simulink model "FourRigidBarsAug"  (R2025b)
settings: Solver=VariableStepAuto  StartTime=0.0  StopTime=10.0  RelTol=1e-3
undefined symbols (not defined in the file): I1_G, I2_G, I3_G, Ignew, InvDynAug, Jr, l1, l2, l3, m1, m2, m3, ra_norm, sig4, Theta, uss
libraries: RCTblocks x99
(part 1 of 2)
settings Model: Creator=d.alazard  LastModifiedBy=andre
settings SolverCC: AlgebraicLoopSolver=TrustRegion
settings OptimizationCC: DefaultParameterBehavior=Inlined  BufferReuse=off
settings DebuggingCC: AlgebraicLoopMsg=none  UnconnectedInputMsg=warning  UnconnectedOutputMsg=warning  UnconnectedLineMsg=warning  InitInArrayFormatMsg=none
settings ModelReferenceCC: EnableRefExpFcnMdlSchedulingChecks=on
settings RTWCC: GPUComputeCapability=3.5  DLArmComputeVersion=19.05

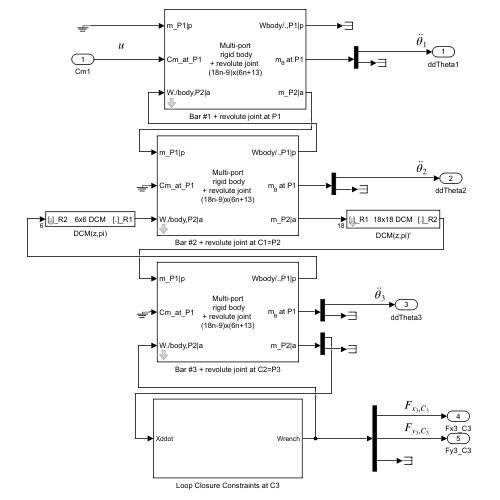
[thumbnail: Simulink's stored preview of the top-level diagram]
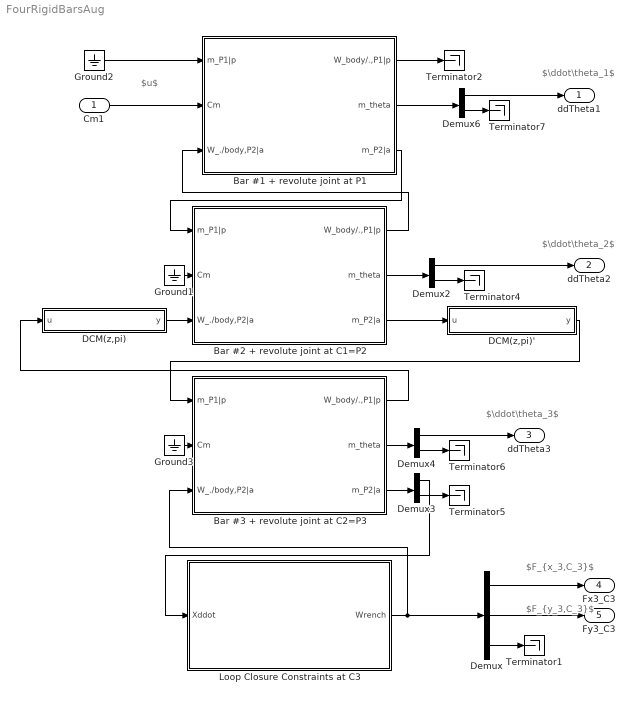
== system FourRigidBarsAug ==
  note: $F_{x_3,C_3}$
  note: $\ddot\theta_1$
  note: $u$
  note: $\ddot\theta_2$
  note: $\ddot\theta_3$
  note: $F_{y_3,C_3}$
  Cm1 : Inport
  Bar #1 + revolute joint at P1 : Subsystem  mask(Multi-port rigid body with revolute joint (18n-9)x(6n+15)){m=m1, Ig=I1_G, OG=[l1/2;0;0], n=2, OP1=[0;0;0], OP2=[l1;0;0], OP3=[0;0;0.25], OP4=[0;12;0], OP5=[0;0;0], ra=[0;0;1], theta=Theta}
      mask prompts: m "Mass (kg)"; Ig "Inertia at G in Ra (kg.m^2)"; OG "OG (3x1 vector in Ra)  (m)"; n "n (number of connection points)"; OP1 "OP1 (3x1 vector in Ra) (m)"; OP2 "OP2 (3x1 vector in Ra) (m)"; OP3 "OP3 (3x1 vector in Ra) (m)"; OP4 "OP4 (3x1 vector in Ra) (m)"; OP5 "OP5 (3x1 vector in Ra) (m)"; ra "ra (joint axis) (3x1 vector)"; theta "Angular configuration (rad)"
      mask help:
      | Computes the (18n-9)x(6n+13) model :
      | - 6x18 transfer from the motion vector to the wrench applied by this body to a parent body at port P1 through a revolute joint,
      | - the 3x1 channel :
      |               * from  the  joint torque applied by the input (parent) shaft to the output (body) shaft
      |               * to the relative motion vector of the output shaft w.r.t the input shaft ([thetaddot;thetadot;theta]),
      | - (n-1) 18x6 transfers from the wrenches applied to this body to the motion vectors at ports P2,P3,..,
      |
      | Input/Output of port P1 are expressed in the parent frame Rp
      | Input/Output of ports P2,P3,... are expressed in the body frame Ra.
      |
      | O: the body reference point
      | G: the center of mass
      | Pi (i=1:n): the n given connection points or ports (n<6).
      | ra: direction of the revolute joint in the Rp (or Ra)
      | theta: angular configuration of the joint (Ra is obtained from Rp by a rotation of theta around ra).
      |
      | All parameters must be expressed in the body frame Ra.
      | Each parameter can be an uncertain parameter declared with the function ureal (except ra)
      |
      | Rk: if "theta" field is: ureal('NAME',0,'Range',[-pi pi])
      | then, ULINEARIZE will provide a model involving the block named "tan_NAME_div4";
      mask init:
      | MultiPortRigidBodyRevAug
      mask Help: web('DocMultiportRigidBodyRevolute.html','-browser')
      mask TypeOptions n: 1 | 2 | 3 | 4 | 5
      mask DialogControl ParameterGroupVar Prompt: Rigid body parameter
      mask DialogControl port1 Prompt: #1
      mask DialogControl port2 Prompt: #2
      mask DialogControl port3 Prompt: #3
      mask DialogControl port4 Prompt: #4
      mask DialogControl port5 Prompt: #5
      mask DialogControl JointParameters Prompt: Revolute joint parameters
      mask Display:
      | disp('Multi-port\n rigid body\n+ revolute joint \n(18n-9)x(6n+13)')
      | 
      | port_label('input', 1,'m_P1|p')
      | port_label('output',1,'Wbody/.,P1|p')
      | port_label('input', 2,'Cm_at_P1')
      | port_label('output',2,'m_\theta at P1','interpreter','tex')
      | 
      | if n>1
      |     for i=2:n
      |         port_label('input', i+1,['W./body,P',num2str(i),'|a'])
      |         port_label('output',i+1,['m_P',num2str(i),'|a'])
      |     end
      | end
  Bar #2 + revolute joint at C1=P2 : Subsystem  mask(Multi-port rigid body with revolute joint (18n-9)x(6n+15)){m=m2, Ig=I2_G, OG=[l2/2;0;0], n=2, OP1=[0;0;0], OP2=[l2;0;0], OP3=[0;0;0.25], OP4=[0;12;0], OP5=[0;0;0], ra=[0;0;-1], theta=Theta}
      mask prompts: m "Mass (kg)"; Ig "Inertia at G in Ra (kg.m^2)"; OG "OG (3x1 vector in Ra)  (m)"; n "n (number of connection points)"; OP1 "OP1 (3x1 vector in Ra) (m)"; OP2 "OP2 (3x1 vector in Ra) (m)"; OP3 "OP3 (3x1 vector in Ra) (m)"; OP4 "OP4 (3x1 vector in Ra) (m)"; OP5 "OP5 (3x1 vector in Ra) (m)"; ra "ra (joint axis) (3x1 vector)"; theta "Angular configuration (rad)"
      mask help:
      | Computes the (18n-9)x(6n+13) model :
      | - 6x18 transfer from the motion vector to the wrench applied by this body to a parent body at port P1 through a revolute joint,
      | - the 3x1 channel :
      |               * from  the  joint torque applied by the input (parent) shaft to the output (body) shaft
      |               * to the relative motion vector of the output shaft w.r.t the input shaft ([thetaddot;thetadot;theta]),
      | - (n-1) 18x6 transfers from the wrenches applied to this body to the motion vectors at ports P2,P3,..,
      |
      | Input/Output of port P1 are expressed in the parent frame Rp
      | Input/Output of ports P2,P3,... are expressed in the body frame Ra.
      |
      | O: the body reference point
      | G: the center of mass
      | Pi (i=1:n): the n given connection points or ports (n<6).
      | ra: direction of the revolute joint in the Rp (or Ra)
      | theta: angular configuration of the joint (Ra is obtained from Rp by a rotation of theta around ra).
      |
      | All parameters must be expressed in the body frame Ra.
      | Each parameter can be an uncertain parameter declared with the function ureal (except ra)
      |
      | Rk: if "theta" field is: ureal('NAME',0,'Range',[-pi pi])
      | then, ULINEARIZE will provide a model involving the block named "tan_NAME_div4";
      mask init:
      | MultiPortRigidBodyRevAug
      mask Help: web('DocMultiportRigidBodyRevolute.html','-browser')
      mask TypeOptions n: 1 | 2 | 3 | 4 | 5
      mask DialogControl ParameterGroupVar Prompt: Rigid body parameter
      mask DialogControl port1 Prompt: #1
      mask DialogControl port2 Prompt: #2
      mask DialogControl port3 Prompt: #3
      mask DialogControl port4 Prompt: #4
      mask DialogControl port5 Prompt: #5
      mask DialogControl JointParameters Prompt: Revolute joint parameters
      mask Display:
      | disp('Multi-port\n rigid body\n+ revolute joint \n(18n-9)x(6n+13)')
      | 
      | port_label('input', 1,'m_P1|p')
      | port_label('output',1,'Wbody/.,P1|p')
      | port_label('input', 2,'Cm_at_P1')
      | port_label('output',2,'m_\theta at P1','interpreter','tex')
      | 
      | if n>1
      |     for i=2:n
      |         port_label('input', i+1,['W./body,P',num2str(i),'|a'])
      |         port_label('output',i+1,['m_P',num2str(i),'|a'])
      |     end
      | end
  Bar #3 + revolute joint at C2=P3 : Subsystem  mask(Multi-port rigid body with revolute joint (18n-9)x(6n+15)){m=m3, Ig=I3_G, OG=[l3/2;0;0], n=2, OP1=[0;0;0], OP2=[l3;0;0], OP3=[0;0;0.25], OP4=[0;12;0], OP5=[0;0;0], ra=[0;0;1], theta=Theta}
      mask prompts: m "Mass (kg)"; Ig "Inertia at G in Ra (kg.m^2)"; OG "OG (3x1 vector in Ra)  (m)"; n "n (number of connection points)"; OP1 "OP1 (3x1 vector in Ra) (m)"; OP2 "OP2 (3x1 vector in Ra) (m)"; OP3 "OP3 (3x1 vector in Ra) (m)"; OP4 "OP4 (3x1 vector in Ra) (m)"; OP5 "OP5 (3x1 vector in Ra) (m)"; ra "ra (joint axis) (3x1 vector)"; theta "Angular configuration (rad)"
      mask help:
      | Computes the (18n-9)x(6n+13) model :
      | - 6x18 transfer from the motion vector to the wrench applied by this body to a parent body at port P1 through a revolute joint,
      | - the 3x1 channel :
      |               * from  the  joint torque applied by the input (parent) shaft to the output (body) shaft
      |               * to the relative motion vector of the output shaft w.r.t the input shaft ([thetaddot;thetadot;theta]),
      | - (n-1) 18x6 transfers from the wrenches applied to this body to the motion vectors at ports P2,P3,..,
      |
      | Input/Output of port P1 are expressed in the parent frame Rp
      | Input/Output of ports P2,P3,... are expressed in the body frame Ra.
      |
      | O: the body reference point
      | G: the center of mass
      | Pi (i=1:n): the n given connection points or ports (n<6).
      | ra: direction of the revolute joint in the Rp (or Ra)
      | theta: angular configuration of the joint (Ra is obtained from Rp by a rotation of theta around ra).
      |
      | All parameters must be expressed in the body frame Ra.
      | Each parameter can be an uncertain parameter declared with the function ureal (except ra)
      |
      | Rk: if "theta" field is: ureal('NAME',0,'Range',[-pi pi])
      | then, ULINEARIZE will provide a model involving the block named "tan_NAME_div4";
      mask init:
      | MultiPortRigidBodyRevAug
      mask Help: web('DocMultiportRigidBodyRevolute.html','-browser')
      mask TypeOptions n: 1 | 2 | 3 | 4 | 5
      mask DialogControl ParameterGroupVar Prompt: Rigid body parameter
      mask DialogControl port1 Prompt: #1
      mask DialogControl port2 Prompt: #2
      mask DialogControl port3 Prompt: #3
      mask DialogControl port4 Prompt: #4
      mask DialogControl port5 Prompt: #5
      mask DialogControl JointParameters Prompt: Revolute joint parameters
      mask Display:
      | disp('Multi-port\n rigid body\n+ revolute joint \n(18n-9)x(6n+13)')
      | 
      | port_label('input', 1,'m_P1|p')
      | port_label('output',1,'Wbody/.,P1|p')
      | port_label('input', 2,'Cm_at_P1')
      | port_label('output',2,'m_\theta at P1','interpreter','tex')
      | 
      | if n>1
      |     for i=2:n
      |         port_label('input', i+1,['W./body,P',num2str(i),'|a'])
      |         port_label('output',i+1,['m_P',num2str(i),'|a'])
      |     end
      | end
  DCM(z,pi) : Subsystem  mask(6x6 Direction cosine matrix (DCM)){rot=[-1 0 0;0 -1 0;0 0 1], transp=off}
      mask prompts: rot "3x3 DCM"; transp "Matrix transposed"
      mask help:
      | For 6 d.o.f. body motion (3 translations and 3 rotations), this block Implement the 6x6 rotation matrix (or its transposed) for a given 3x3 DCM.
      |
      | Considering 2 frames R1 and  R2, the DCM between R1 and R2 is defined as the 3x3 matrix where each column is the component vector of each R2 orthogonal unit vector expressed in R1. Thus
      |
      |    [v]_R1 = DCM  * [v]_R2.
      mask init:
      | if transp,
      |     rot=rot';
      | end
      mask Help: web('Doc6dcm.html','-browser')
      mask Display:
      | disp('6x6 DCM')
      | if transp
      |     port_label('input', 1, '[.]_R1')
      |     port_label('output', 1, '[.]_R2')
      | else
      |     port_label('input', 1, '[.]_R2')
      |     port_label('output', 1, '[.]_R1')
      | end
  DCM(z,pi)' : Subsystem  mask(18x18 Direction cosine matrix (DCM)){rot=[-1 0 0;0 -1 0;0 0 1], transp=on}
      mask prompts: rot "3x3 DCM"; transp "Matrix transposed"
      mask help:
      | For 6 d.o.f. body motion vector (3 translations and 3 rotations, accelerations, velocities and positions), this block Implement the 18x18 rotation matrix (or its transposed) for a given 3x3 DCM.
      |
      | Considering 2 frames R1 and  R2, the DCM between R1 and R2 is defined as the 3x3 matrix where each column is the component vector of each R2 orthogonal unit vector expressed in R1. Thus
      |
      |    [v]_R1 = DCM  * [v]_R2.
      mask init:
      | if transp,
      |     rot=rot';
      | end
      mask Help: web('Doc18dcm.html','-browser')
      mask Display:
      | disp('18x18 DCM')
      | if transp
      |     port_label('input', 1, '[.]_R1')
      |     port_label('output', 1, '[.]_R2')
      | else
      |     port_label('input', 1, '[.]_R2')
      |     port_label('output', 1, '[.]_R1')
      | end
  Demux : Demux  Outputs=[1 1 4]
  Demux2 : Demux  Outputs=[1 2]
  Demux3 : Demux  Outputs=[6 12]
  Demux4 : Demux  Outputs=[1 2]
  Demux6 : Demux  Outputs=[1 2]
  Ground1 : Ground
  Ground2 : Ground
  Ground3 : Ground
  Loop Closure Constraints at C3 : Subsystem
  Terminator{1..2,4..7} (6 alike) : Terminator
  ddTheta1 : Outport
  ddTheta2 : Outport  Port=2
  ddTheta3 : Outport  Port=3
  Fx3_C3 : Outport  Port=4
  Fy3_C3 : Outport  Port=5
  wires:
  Bar #2 + revolute joint at C1=P2/1(W_body/.,P1|p) -> Bar #1 + revolute joint at P1/3(W_./body,P2|a)
  Cm1/1 -> Bar #1 + revolute joint at P1/2(Cm)
  Ground1/1 -> Bar #2 + revolute joint at C1=P2/2(Cm)
  Demux6/1 -> ddTheta1/1
  Demux2/1 -> ddTheta2/1
  DCM(z,pi)/1(y) -> Bar #2 + revolute joint at C1=P2/3(W_./body,P2|a)
  DCM(z,pi)'/1(y) -> Bar #3 + revolute joint at C2=P3/1(m_P1|p)
  Bar #3 + revolute joint at C2=P3/1(W_body/.,P1|p) -> DCM(z,pi)/1(u)
  Ground3/1 -> Bar #3 + revolute joint at C2=P3/2(Cm)
  Ground2/1 -> Bar #1 + revolute joint at P1/1(m_P1|p)
  Bar #1 + revolute joint at P1/1(W_body/.,P1|p) -> Terminator2/1
  Demux3/1 -> Loop Closure Constraints at C3/1(Xddot)
  Loop Closure Constraints at C3/1(Wrench) -> Demux/1, Bar #3 + revolute joint at C2=P3/3(W_./body,P2|a)
  Demux/3 -> Terminator1/1
  Demux/1 -> Fx3_C3/1
  Demux/2 -> Fy3_C3/1
  Bar #2 + revolute joint at C1=P2/2(m_theta) -> Demux2/1
  Demux2/2 -> Terminator4/1
  Demux4/2 -> Terminator6/1
  Bar #3 + revolute joint at C2=P3/2(m_theta) -> Demux4/1
  Demux3/2 -> Terminator5/1
  Bar #3 + revolute joint at C2=P3/3(m_P2|a) -> Demux3/1
  Demux4/1 -> ddTheta3/1
  Demux6/2 -> Terminator7/1
  Bar #1 + revolute joint at P1/2(m_theta) -> Demux6/1
  Bar #1 + revolute joint at P1/3(m_P2|a) -> Bar #2 + revolute joint at C1=P2/1(m_P1|p)
  Bar #2 + revolute joint at C1=P2/3(m_P2|a) -> DCM(z,pi)'/1(u)

== system FourRigidBarsAug/Bar #1 + revolute joint at P1 ==
  m_P1|p : Inport
  Cm : Inport  Port=2
  W_./body,P2|a : Inport  Port=3
  Multi port rigid body : Subsystem  mask(Multi-port rigid body (6nx6n)){m=m, Ig=Ignew, OG=OG, n=2, numinv=1, OP1=[0;0;0], OP2=[l1;0;0], OP3=[0;0;0.25], OP4=[0;12;0], OP5=[0;0;0]}
      mask prompts: m "Mass (Kg)"; Ig "Inertia (at G, Kg m^2)"; OG "OG (3x1 vector, m)"; n "Number of ports"; numinv "Port to be inverted"; OP1 "OP1 (3x1 vector, m)"; OP2 "OP2 (3x1 vector, m)"; OP3 "OP3 (3x1 vector, m)"; OP4 "OP4 (3x1 vector, m)"; OP5 "OP5 (3x1 vector,m)"
      mask help:
      | 6nx6n dynamic model of a rigid body at n given points (ports) between wrenches applied at the n points (input) and acceleration twists at these points (output).
      |
      | 0: the reference point
      | G: the center of mass
      | Pi (i=1:n): the n given connection points (n<6).
      |
      | All parameters are expressed in the body frame.
      | Each parameter can be an uncertain parameter declared with "ureal"
      |
      | The 6x6 channel associated to one port can be inverted: then the input of this channel is the acceleration twist imposed at this point and the output is the wrench applied by this body.
      mask init:
      | MultiPortRigidBodyAug
      mask Help: web('Docmultiportrigidbody.html','-browser')
      mask TypeOptions n: 1 | 2 | 3 | 4 | 5
      mask TypeOptions numinv: 1 | 2 | 3 | 4 | 5
      mask DialogControl ParameterGroupVar Prompt: Main parameters
      mask DialogControl port1 Prompt: Port #1
      mask DialogControl port2 Prompt: #2
      mask DialogControl port3 Prompt: #3
      mask DialogControl port4 Prompt: #4
      mask DialogControl port5 Prompt: #5
      mask Display:
      | disp('Multi-port\n rigid body\n [18(n-1)+6]x[6(n-1)+18])')
      | if n==1,
      |     if numinv==1,
      |         port_label('input', 1,'m_P')
      |         port_label('output',1,'W_body/.,P')
      |     else
      |         port_label('input', 1,'W_./body,P')
      |         port_label('output',1,'m_P')
      |     end
      | else
      |     for ii=1:n
      |         if numinv==ii,
      |             port_label('output',ii,['W_body/.,P',num2str(ii)])
      |             port_label('input', ii,['m_P',num2str(ii)])
      |         else
      |             port_label('input', ii,['W_./body,P',num2str(ii)])
      |             port_label('output',ii,['m_P',num2str(ii)])
      |         end
      |     end
      | end
  Revolute joint + configuration : Subsystem  mask(Revolute joint){ra=ra_norm, Jr=Jr, theta=theta}
      mask prompts: ra "Direction of the joint in the local frame (3x1 vector)"; Jr "Rotor inertia (kg.m^2)"; theta "Angular configuration (rad)"
      mask help:
      | This block implement the TITOP model of of a revolute joint.
      | The last channel is the transfer between the torque applied inside the joint by the input shaft to the output shaft and the relative angular acceleration of the output shaft w.r.t the input shaft.
      |
      | Angular configuration can be a vayring parameter: Ex:
      | ureal('NAME',0,'Range',[-pi pi])
      |
      | Then, ULINEARIZE will provide a model involving the block named "tan_NAME_div4";
      mask init:
      | pass=ra2DCMi(ra);
      | ran=[ra(1);ra(2);ra(3)]/norm(ra);
      mask Help: web('DocRevoluteJoint_configuration.html','-browser')
      mask Display:
      | disp('Revolute joint\nTITOP model\n+ angle configuration')
      | port_label('input', 1, 'W_./r_out|a')
      | port_label('output', 1, 'm_out|a')
      | port_label('input', 2, 'm_in|p')
      | port_label('output', 2, 'W_r_in/.|p')
      | port_label('input', 3, 'Cm')
      | port_label('output', 3, 'm_\theta','interpreter','tex')
  W_body/.,P1|p : Outport  VectorParamsAs1DForOutWhenUnconnected=off
  m_theta : Outport  Port=2  VectorParamsAs1DForOutWhenUnconnected=off
  m_P2|a : Outport  Port=3
  wires:
  Revolute joint + configuration/1(m_out|a) -> Multi port rigid body/1(in1)
  Multi port rigid body/1(out1) -> Revolute joint + configuration/1(W_./r_out|a)
  m_P1|p/1 -> Revolute joint + configuration/2(m_in|p)
  Cm/1 -> Revolute joint + configuration/3(Cm)
  Revolute joint + configuration/2(W_r_in/.|p) -> W_body/.,P1|p/1
  Revolute joint + configuration/3(m_theta) -> m_theta/1
  W_./body,P2|a/1 -> Multi port rigid body/2(in2)
  Multi port rigid body/2(out2) -> m_P2|a/1

== system FourRigidBarsAug/Bar #2 + revolute joint at C1=P2 ==
  m_P1|p : Inport
  Cm : Inport  Port=2
  W_./body,P2|a : Inport  Port=3
  Multi port rigid body : Subsystem  mask(Multi-port rigid body (6nx6n)){m=m, Ig=Ignew, OG=OG, n=2, numinv=1, OP1=[0;0;0], OP2=[l2;0;0], OP3=[0;0;0.25], OP4=[0;12;0], OP5=[0;0;0]}
      mask prompts: m "Mass (Kg)"; Ig "Inertia (at G, Kg m^2)"; OG "OG (3x1 vector, m)"; n "Number of ports"; numinv "Port to be inverted"; OP1 "OP1 (3x1 vector, m)"; OP2 "OP2 (3x1 vector, m)"; OP3 "OP3 (3x1 vector, m)"; OP4 "OP4 (3x1 vector, m)"; OP5 "OP5 (3x1 vector,m)"
      mask help:
      | 6nx6n dynamic model of a rigid body at n given points (ports) between wrenches applied at the n points (input) and acceleration twists at these points (output).
      |
      | 0: the reference point
      | G: the center of mass
      | Pi (i=1:n): the n given connection points (n<6).
      |
      | All parameters are expressed in the body frame.
      | Each parameter can be an uncertain parameter declared with "ureal"
      |
      | The 6x6 channel associated to one port can be inverted: then the input of this channel is the acceleration twist imposed at this point and the output is the wrench applied by this body.
      mask init:
      | MultiPortRigidBodyAug
      mask Help: web('Docmultiportrigidbody.html','-browser')
      mask TypeOptions n: 1 | 2 | 3 | 4 | 5
      mask TypeOptions numinv: 1 | 2 | 3 | 4 | 5
      mask DialogControl ParameterGroupVar Prompt: Main parameters
      mask DialogControl port1 Prompt: Port #1
      mask DialogControl port2 Prompt: #2
      mask DialogControl port3 Prompt: #3
      mask DialogControl port4 Prompt: #4
      mask DialogControl port5 Prompt: #5
      mask Display:
      | disp('Multi-port\n rigid body\n [18(n-1)+6]x[6(n-1)+18])')
      | if n==1,
      |     if numinv==1,
      |         port_label('input', 1,'m_P')
      |         port_label('output',1,'W_body/.,P')
      |     else
      |         port_label('input', 1,'W_./body,P')
      |         port_label('output',1,'m_P')
      |     end
      | else
      |     for ii=1:n
      |         if numinv==ii,
      |             port_label('output',ii,['W_body/.,P',num2str(ii)])
      |             port_label('input', ii,['m_P',num2str(ii)])
      |         else
      |             port_label('input', ii,['W_./body,P',num2str(ii)])
      |             port_label('output',ii,['m_P',num2str(ii)])
      |         end
      |     end
      | end
  Revolute joint + configuration : Subsystem  mask(Revolute joint){ra=ra_norm, Jr=Jr, theta=theta}
      mask prompts: ra "Direction of the joint in the local frame (3x1 vector)"; Jr "Rotor inertia (kg.m^2)"; theta "Angular configuration (rad)"
      mask help:
      | This block implement the TITOP model of of a revolute joint.
      | The last channel is the transfer between the torque applied inside the joint by the input shaft to the output shaft and the relative angular acceleration of the output shaft w.r.t the input shaft.
      |
      | Angular configuration can be a vayring parameter: Ex:
      | ureal('NAME',0,'Range',[-pi pi])
      |
      | Then, ULINEARIZE will provide a model involving the block named "tan_NAME_div4";
      mask init:
      | pass=ra2DCMi(ra);
      | ran=[ra(1);ra(2);ra(3)]/norm(ra);
      mask Help: web('DocRevoluteJoint_configuration.html','-browser')
      mask Display:
      | disp('Revolute joint\nTITOP model\n+ angle configuration')
      | port_label('input', 1, 'W_./r_out|a')
      | port_label('output', 1, 'm_out|a')
      | port_label('input', 2, 'm_in|p')
      | port_label('output', 2, 'W_r_in/.|p')
      | port_label('input', 3, 'Cm')
      | port_label('output', 3, 'm_\theta','interpreter','tex')
  W_body/.,P1|p : Outport  VectorParamsAs1DForOutWhenUnconnected=off
  m_theta : Outport  Port=2  VectorParamsAs1DForOutWhenUnconnected=off
  m_P2|a : Outport  Port=3
  wires:
  Revolute joint + configuration/1(m_out|a) -> Multi port rigid body/1(in1)
  Multi port rigid body/1(out1) -> Revolute joint + configuration/1(W_./r_out|a)
  m_P1|p/1 -> Revolute joint + configuration/2(m_in|p)
  Cm/1 -> Revolute joint + configuration/3(Cm)
  Revolute joint + configuration/2(W_r_in/.|p) -> W_body/.,P1|p/1
  Revolute joint + configuration/3(m_theta) -> m_theta/1
  W_./body,P2|a/1 -> Multi port rigid body/2(in2)
  Multi port rigid body/2(out2) -> m_P2|a/1

== system FourRigidBarsAug/Bar #3 + revolute joint at C2=P3 ==
  m_P1|p : Inport
  Cm : Inport  Port=2
  W_./body,P2|a : Inport  Port=3
  Multi port rigid body : Subsystem  mask(Multi-port rigid body (6nx6n)){m=m, Ig=Ignew, OG=OG, n=2, numinv=1, OP1=[0;0;0], OP2=[l3;0;0], OP3=[0;0;0.25], OP4=[0;12;0], OP5=[0;0;0]}
      mask prompts: m "Mass (Kg)"; Ig "Inertia (at G, Kg m^2)"; OG "OG (3x1 vector, m)"; n "Number of ports"; numinv "Port to be inverted"; OP1 "OP1 (3x1 vector, m)"; OP2 "OP2 (3x1 vector, m)"; OP3 "OP3 (3x1 vector, m)"; OP4 "OP4 (3x1 vector, m)"; OP5 "OP5 (3x1 vector,m)"
      mask help:
      | 6nx6n dynamic model of a rigid body at n given points (ports) between wrenches applied at the n points (input) and acceleration twists at these points (output).
      |
      | 0: the reference point
      | G: the center of mass
      | Pi (i=1:n): the n given connection points (n<6).
      |
      | All parameters are expressed in the body frame.
      | Each parameter can be an uncertain parameter declared with "ureal"
      |
      | The 6x6 channel associated to one port can be inverted: then the input of this channel is the acceleration twist imposed at this point and the output is the wrench applied by this body.
      mask init:
      | MultiPortRigidBodyAug
      mask Help: web('Docmultiportrigidbody.html','-browser')
      mask TypeOptions n: 1 | 2 | 3 | 4 | 5
      mask TypeOptions numinv: 1 | 2 | 3 | 4 | 5
      mask DialogControl ParameterGroupVar Prompt: Main parameters
      mask DialogControl port1 Prompt: Port #1
      mask DialogControl port2 Prompt: #2
      mask DialogControl port3 Prompt: #3
      mask DialogControl port4 Prompt: #4
      mask DialogControl port5 Prompt: #5
      mask Display:
      | disp('Multi-port\n rigid body\n [18(n-1)+6]x[6(n-1)+18])')
      | if n==1,
      |     if numinv==1,
      |         port_label('input', 1,'m_P')
      |         port_label('output',1,'W_body/.,P')
      |     else
      |         port_label('input', 1,'W_./body,P')
      |         port_label('output',1,'m_P')
      |     end
      | else
      |     for ii=1:n
      |         if numinv==ii,
      |             port_label('output',ii,['W_body/.,P',num2str(ii)])
      |             port_label('input', ii,['m_P',num2str(ii)])
      |         else
      |             port_label('input', ii,['W_./body,P',num2str(ii)])
      |             port_label('output',ii,['m_P',num2str(ii)])
      |         end
      |     end
      | end
  Revolute joint + configuration : Subsystem  mask(Revolute joint){ra=ra_norm, Jr=Jr, theta=theta}
      mask prompts: ra "Direction of the joint in the local frame (3x1 vector)"; Jr "Rotor inertia (kg.m^2)"; theta "Angular configuration (rad)"
      mask help:
      | This block implement the TITOP model of of a revolute joint.
      | The last channel is the transfer between the torque applied inside the joint by the input shaft to the output shaft and the relative angular acceleration of the output shaft w.r.t the input shaft.
      |
      | Angular configuration can be a vayring parameter: Ex:
      | ureal('NAME',0,'Range',[-pi pi])
      |
      | Then, ULINEARIZE will provide a model involving the block named "tan_NAME_div4";
      mask init:
      | pass=ra2DCMi(ra);
      | ran=[ra(1);ra(2);ra(3)]/norm(ra);
      mask Help: web('DocRevoluteJoint_configuration.html','-browser')
      mask Display:
      | disp('Revolute joint\nTITOP model\n+ angle configuration')
      | port_label('input', 1, 'W_./r_out|a')
      | port_label('output', 1, 'm_out|a')
      | port_label('input', 2, 'm_in|p')
      | port_label('output', 2, 'W_r_in/.|p')
      | port_label('input', 3, 'Cm')
      | port_label('output', 3, 'm_\theta','interpreter','tex')
  W_body/.,P1|p : Outport  VectorParamsAs1DForOutWhenUnconnected=off
  m_theta : Outport  Port=2  VectorParamsAs1DForOutWhenUnconnected=off
  m_P2|a : Outport  Port=3
  wires:
  Revolute joint + configuration/1(m_out|a) -> Multi port rigid body/1(in1)
  Multi port rigid body/1(out1) -> Revolute joint + configuration/1(W_./r_out|a)
  m_P1|p/1 -> Revolute joint + configuration/2(m_in|p)
  Cm/1 -> Revolute joint + configuration/3(Cm)
  Revolute joint + configuration/2(W_r_in/.|p) -> W_body/.,P1|p/1
  Revolute joint + configuration/3(m_theta) -> m_theta/1
  W_./body,P2|a/1 -> Multi port rigid body/2(in2)
  Multi port rigid body/2(out2) -> m_P2|a/1

== system FourRigidBarsAug/DCM(z,pi) ==
  u : Inport  PortDimensions=6
  Demux : Demux  Outputs=[3 3]
  Mux : Mux  Inputs=[3 3]
  rotation : Gain  Gain=rot  Multiplication=Matrix(K*u) (u vector)
  translation : Gain  Gain=rot  Multiplication=Matrix(K*u) (u vector)
  y : Outport  VectorParamsAs1DForOutWhenUnconnected=off
  wires:
  rotation/1 -> Mux/2
  translation/1 -> Mux/1
  Demux/1 -> translation/1
  u/1 -> Demux/1
  Mux/1 -> y/1
  Demux/2 -> rotation/1

== system FourRigidBarsAug/DCM(z,pi)' ==
  u : Inport  PortDimensions=18
  Demux : Demux  Outputs=[3 3 3 3 3 3]
  Mux : Mux  Inputs=[3 3 3 3 3 3]
  rotation : Gain  Gain=rot  Multiplication=Matrix(K*u) (u vector)
  rotation1 : Gain  Gain=rot  Multiplication=Matrix(K*u) (u vector)
  rotation2 : Gain  Gain=rot  Multiplication=Matrix(K*u) (u vector)
  translation : Gain  Gain=rot  Multiplication=Matrix(K*u) (u vector)
  translation1 : Gain  Gain=rot  Multiplication=Matrix(K*u) (u vector)
  translation2 : Gain  Gain=rot  Multiplication=Matrix(K*u) (u vector)
  y : Outport  VectorParamsAs1DForOutWhenUnconnected=off
  wires:
  Demux/6 -> rotation2/1
  rotation2/1 -> Mux/6
  translation2/1 -> Mux/5
  Demux/5 -> translation2/1
  rotation1/1 -> Mux/4
  translation1/1 -> Mux/3
  Demux/3 -> translation1/1
  Demux/4 -> rotation1/1
  Demux/2 -> rotation/1
  Mux/1 -> y/1
  u/1 -> Demux/1
  Demux/1 -> translation/1
  translation/1 -> Mux/1
  rotation/1 -> Mux/2

== system FourRigidBarsAug/Loop Closure Constraints at C3 ==
  Xddot : Inport
  Demux : Demux  Outputs=6
  Ground{5..8} (4 alike) : Ground
  Mux : Mux  Inputs=6
  Terminator{1,3..5} (4 alike) : Terminator
  mx : Gain  Gain=-1e6
  my : Gain  Gain=-1e6
  Wrench : Outport
  wires:
  Ground7/1 -> Mux/5
  Ground6/1 -> Mux/4
  Xddot/1 -> Demux/1
  Demux/4 -> Terminator3/1
  Ground8/1 -> Mux/6
  Demux/6 -> Terminator5/1
  Demux/5 -> Terminator4/1
  mx/1 -> Mux/1
  Demux/3 -> Terminator1/1
  my/1 -> Mux/2
  Mux/1 -> Wrench/1
  Ground5/1 -> Mux/3
  Demux/1 -> mx/1
  Demux/2 -> my/1

== system FourRigidBarsAug/Bar #1 + revolute joint at P1/Multi port rigid body ==
  in1 : Inport  PortDimensions=18
  in2 : Inport  Port=2  PortDimensions=6
  Demux : Demux  Outputs=[ 6 18]
  Gain : RCTblocks/Uncertain State Space  Tag=USS  USystem=uss(InvDynAug)  UValue=[]  X0=[]  uX0=[]
  Mux : Mux  Inputs=[ 18 6]
  out1 : Outport
  out2 : Outport  Port=2
  wires:
  Demux/2 -> out2/1
  in2/1 -> Mux/2
  Demux/1 -> out1/1
  in1/1 -> Mux/1
  Gain/1 -> Demux/1
  Mux/1 -> Gain/1

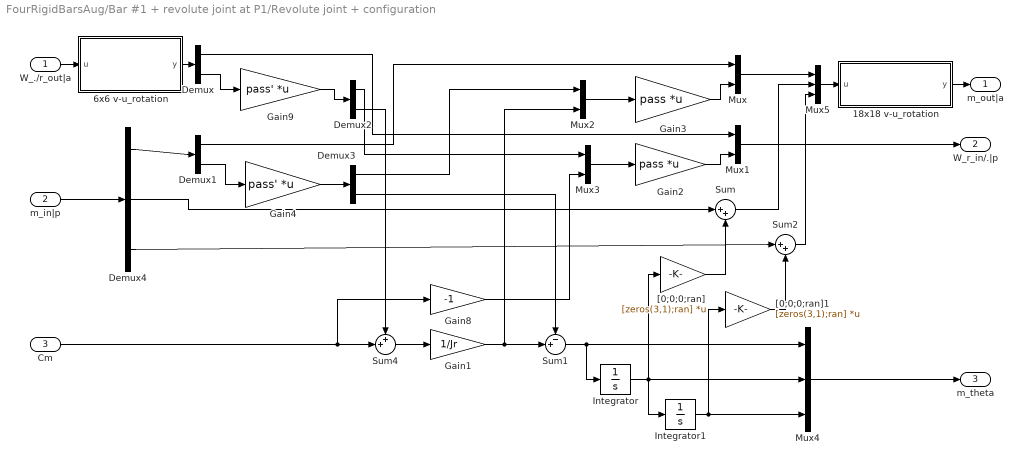
== system FourRigidBarsAug/Bar #1 + revolute joint at P1/Revolute joint + configuration ==
  W_./r_out|a : Inport  PortDimensions=6
  m_in|p : Inport  Port=2  PortDimensions=18
  Cm : Inport  Port=3  PortDimensions=1
  18x18 v-u_rotation : Subsystem  mask(18x18 rotation matrix (around a given axis)){ra=ra, theta=theta, transp=on}
      mask prompts: ra "Rotation axis (3x1 vector)"; theta "Angle (rad)"; transp "Matrix transposed"
      mask help:
      | For 6 d.o.f. body motion vector (3 translations and 3 rotations, acceleration velocities and positions), this block Implement the 18x18 rotation matrix (or its transposed)  for a given angle around a given axis.
      |
      | Angle  (rad) can be an uncertain parameter declared with "ureal" with mode 'Range'
      | Ex: ureal('NAME',0,'Range',[-pi pi])
      | Then, ULINEARIZE will provide a model involving the block named "tan_NAME_div4".
      mask init:
      | vUrotation3x3
      mask Help: web('Doc6vurotation.html','-browser')
      mask Display:
      | disp('v-rot\n18x18')
      | if transp
      |     port_label('input', 1, '[.]_R1')
      |     port_label('output', 1, '[.]_R2')
      | else
      |     port_label('input', 1, '[.]_R2')
      |     port_label('output', 1, '[.]_R1')
      | end
  6x6 v-u_rotation : Subsystem  mask(6x6 rotation matrix (around a given axis)){ra=ra, theta=theta, transp=off}
      mask prompts: ra "Rotation axis (3x1 vector)"; theta "Angle (rad)"; transp "Matrix transposed"
      mask help:
      | For 6 d.o.f. body motion (3 translations and 3 rotations), this block Implement the 6x6 rotation matrix (or its transposed) for a given angle around a given axis.
      |
      | Angle  (rad) can be an uncertain parameter declared with "ureal" with mode 'Range'
      | Ex: ureal('NAME',0,'Range',[-pi pi])
      | Then, ULINEARIZE will provide a model involving the block named "tan_NAME_div4".
      mask init:
      | vUrotation3x3
      mask Help: web('Doc6vurotation.html','-browser')
      mask Display:
      | disp('v-rot\n6x6')
      | if transp
      |     port_label('input', 1, '[.]_R1')
      |     port_label('output', 1, '[.]_R2')
      | else
      |     port_label('input', 1, '[.]_R2')
      |     port_label('output', 1, '[.]_R1')
      | end
  Demux : Demux  Outputs=[3 3]
  Demux1 : Demux  Outputs=[3 3]
  Demux2 : Demux  Outputs=[2 1]
  Demux3 : Demux  Outputs=[2 1]
  Demux4 : Demux  Outputs=[6 6 6]
  Gain1 : Gain  Gain=1/Jr
  Gain2 : Gain  Gain=pass  Multiplication=Matrix(K*u) (u vector)
  Gain3 : Gain  Gain=pass  Multiplication=Matrix(K*u) (u vector)
  Gain4 : Gain  Gain=pass'  Multiplication=Matrix(K*u) (u vector)
  Gain8 : Gain  Gain=-1
  Gain9 : Gain  Gain=pass'  Multiplication=Matrix(K*u) (u vector)
  Integrator : Integrator
  Integrator1 : Integrator
  Mux : Mux  Inputs=[3 3]
  Mux1 : Mux  Inputs=[3 3]
  Mux2 : Mux  Inputs=[2 1]
  Mux3 : Mux  Inputs=[2 1]
  Mux4 : Mux  Inputs=3
  Mux5 : Mux  Inputs=[6 6 6]
  Sum : Sum  Inputs=|++
  Sum1 : Sum  Inputs=-+|
  Sum2 : Sum  Inputs=|++
  Sum4 : Sum  Inputs=++|
  "[0;0;0;ran]" : Gain  Gain=[zeros(3,1);ran]  Multiplication=Matrix(K*u) (u vector)
  "[0;0;0;ran]1" : Gain  Gain=[zeros(3,1);ran]  Multiplication=Matrix(K*u) (u vector)
  m_out|a : Outport  VectorParamsAs1DForOutWhenUnconnected=off
  W_r_in/.|p : Outport  Port=2  VectorParamsAs1DForOutWhenUnconnected=off
  m_theta : Outport  Port=3  VectorParamsAs1DForOutWhenUnconnected=off
  wires:
  18x18 v-u_rotation/1(y) -> m_out|a/1
  6x6 v-u_rotation/1(y) -> Demux/1
  Demux3/1 -> Mux2/1
  Demux2/1 -> Mux3/1
  Gain8/1 -> Mux3/2
  Mux3/1 -> Gain2/1
  Gain4/1 -> Demux3/1
  Demux1/2 -> Gain4/1
  Mux2/1 -> Gain3/1
  Demux2/2 -> Sum4/1
  Gain9/1 -> Demux2/1
  Demux3/2 -> Sum1/1
  Gain3/1 -> Mux/2
  Sum4/1 -> Gain1/1
  Gain1/1 -> Sum1/2, Mux2/2
  Demux/2 -> Gain9/1
  Gain2/1 -> Mux1/2
  Demux/1 -> Mux1/1
  Cm/1 -> Sum4/2, Gain8/1
  Demux1/1 -> Mux/1
  Mux1/1 -> W_r_in/.|p/1
  W_./r_out|a/1 -> 6x6 v-u_rotation/1(u)
  Demux4/1 -> Demux1/1
  m_in|p/1 -> Demux4/1
  Integrator/1 -> "[0;0;0;ran]"/1, Mux4/2, Integrator1/1
  Mux4/1 -> m_theta/1
  Sum1/1 -> Integrator/1, Mux4/1
  Integrator1/1 -> "[0;0;0;ran]1"/1, Mux4/3
  "[0;0;0;ran]"/1 -> Sum/2
  "[0;0;0;ran]1"/1 -> Sum2/2
  Demux4/2 -> Sum/1
  Demux4/3 -> Sum2/1
  Mux/1 -> Mux5/1
  Mux5/1 -> 18x18 v-u_rotation/1(u)
  Sum/1 -> Mux5/2
  Sum2/1 -> Mux5/3

== system FourRigidBarsAug/Bar #2 + revolute joint at C1=P2/Multi port rigid body ==
  in1 : Inport  PortDimensions=18
  in2 : Inport  Port=2  PortDimensions=6
  Demux : Demux  Outputs=[ 6 18]
  Gain : RCTblocks/Uncertain State Space  Tag=USS  USystem=uss(InvDynAug)  UValue=[]  X0=[]  uX0=[]
  Mux : Mux  Inputs=[ 18 6]
  out1 : Outport
  out2 : Outport  Port=2
  wires:
  Mux/1 -> Gain/1
  Gain/1 -> Demux/1
  in1/1 -> Mux/1
  Demux/1 -> out1/1
  in2/1 -> Mux/2
  Demux/2 -> out2/1

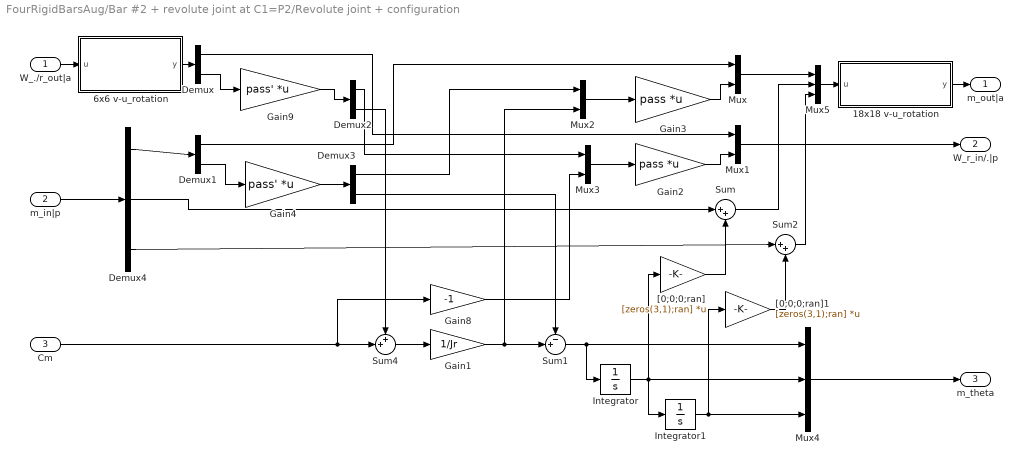
== system FourRigidBarsAug/Bar #2 + revolute joint at C1=P2/Revolute joint + configuration ==
  W_./r_out|a : Inport  PortDimensions=6
  m_in|p : Inport  Port=2  PortDimensions=18
  Cm : Inport  Port=3  PortDimensions=1
  18x18 v-u_rotation : Subsystem  mask(18x18 rotation matrix (around a given axis)){ra=ra, theta=theta, transp=on}
      mask prompts: ra "Rotation axis (3x1 vector)"; theta "Angle (rad)"; transp "Matrix transposed"
      mask help:
      | For 6 d.o.f. body motion vector (3 translations and 3 rotations, acceleration velocities and positions), this block Implement the 18x18 rotation matrix (or its transposed)  for a given angle around a given axis.
      |
      | Angle  (rad) can be an uncertain parameter declared with "ureal" with mode 'Range'
      | Ex: ureal('NAME',0,'Range',[-pi pi])
      | Then, ULINEARIZE will provide a model involving the block named "tan_NAME_div4".
      mask init:
      | vUrotation3x3
      mask Help: web('Doc6vurotation.html','-browser')
      mask Display:
      | disp('v-rot\n18x18')
      | if transp
      |     port_label('input', 1, '[.]_R1')
      |     port_label('output', 1, '[.]_R2')
      | else
      |     port_label('input', 1, '[.]_R2')
      |     port_label('output', 1, '[.]_R1')
      | end
  6x6 v-u_rotation : Subsystem  mask(6x6 rotation matrix (around a given axis)){ra=ra, theta=theta, transp=off}
      mask prompts: ra "Rotation axis (3x1 vector)"; theta "Angle (rad)"; transp "Matrix transposed"
      mask help:
      | For 6 d.o.f. body motion (3 translations and 3 rotations), this block Implement the 6x6 rotation matrix (or its transposed) for a given angle around a given axis.
      |
      | Angle  (rad) can be an uncertain parameter declared with "ureal" with mode 'Range'
      | Ex: ureal('NAME',0,'Range',[-pi pi])
      | Then, ULINEARIZE will provide a model involving the block named "tan_NAME_div4".
      mask init:
      | vUrotation3x3
      mask Help: web('Doc6vurotation.html','-browser')
      mask Display:
      | disp('v-rot\n6x6')
      | if transp
      |     port_label('input', 1, '[.]_R1')
      |     port_label('output', 1, '[.]_R2')
      | else
      |     port_label('input', 1, '[.]_R2')
      |     port_label('output', 1, '[.]_R1')
      | end
  Demux : Demux  Outputs=[3 3]
  Demux1 : Demux  Outputs=[3 3]
  Demux2 : Demux  Outputs=[2 1]
  Demux3 : Demux  Outputs=[2 1]
  Demux4 : Demux  Outputs=[6 6 6]
  Gain1 : Gain  Gain=1/Jr
  Gain2 : Gain  Gain=pass  Multiplication=Matrix(K*u) (u vector)
  Gain3 : Gain  Gain=pass  Multiplication=Matrix(K*u) (u vector)
  Gain4 : Gain  Gain=pass'  Multiplication=Matrix(K*u) (u vector)
  Gain8 : Gain  Gain=-1
  Gain9 : Gain  Gain=pass'  Multiplication=Matrix(K*u) (u vector)
  Integrator : Integrator
  Integrator1 : Integrator
  Mux : Mux  Inputs=[3 3]
  Mux1 : Mux  Inputs=[3 3]
  Mux2 : Mux  Inputs=[2 1]
  Mux3 : Mux  Inputs=[2 1]
  Mux4 : Mux  Inputs=3
  Mux5 : Mux  Inputs=[6 6 6]
  Sum : Sum  Inputs=|++
  Sum1 : Sum  Inputs=-+|
  Sum2 : Sum  Inputs=|++
  Sum4 : Sum  Inputs=++|
  "[0;0;0;ran]" : Gain  Gain=[zeros(3,1);ran]  Multiplication=Matrix(K*u) (u vector)
  "[0;0;0;ran]1" : Gain  Gain=[zeros(3,1);ran]  Multiplication=Matrix(K*u) (u vector)
  m_out|a : Outport  VectorParamsAs1DForOutWhenUnconnected=off
  W_r_in/.|p : Outport  Port=2  VectorParamsAs1DForOutWhenUnconnected=off
  m_theta : Outport  Port=3  VectorParamsAs1DForOutWhenUnconnected=off
  wires:
  Sum2/1 -> Mux5/3
  Sum/1 -> Mux5/2
  Mux5/1 -> 18x18 v-u_rotation/1(u)
  Mux/1 -> Mux5/1
  Demux4/3 -> Sum2/1
  Demux4/2 -> Sum/1
  "[0;0;0;ran]1"/1 -> Sum2/2
  "[0;0;0;ran]"/1 -> Sum/2
  Integrator1/1 -> Mux4/3, "[0;0;0;ran]1"/1
  Sum1/1 -> Mux4/1, Integrator/1
  Mux4/1 -> m_theta/1
  Integrator/1 -> Integrator1/1, Mux4/2, "[0;0;0;ran]"/1
  m_in|p/1 -> Demux4/1
  Demux4/1 -> Demux1/1
  W_./r_out|a/1 -> 6x6 v-u_rotation/1(u)
  Mux1/1 -> W_r_in/.|p/1
  Demux1/1 -> Mux/1
  Cm/1 -> Gain8/1, Sum4/2
  Demux/1 -> Mux1/1
  Gain2/1 -> Mux1/2
  Demux/2 -> Gain9/1
  Gain1/1 -> Mux2/2, Sum1/2
  Sum4/1 -> Gain1/1
  Gain3/1 -> Mux/2
  Demux3/2 -> Sum1/1
  Gain9/1 -> Demux2/1
  Demux2/2 -> Sum4/1
  Mux2/1 -> Gain3/1
  Demux1/2 -> Gain4/1
  Gain4/1 -> Demux3/1
  Mux3/1 -> Gain2/1
  Gain8/1 -> Mux3/2
  Demux2/1 -> Mux3/1
  Demux3/1 -> Mux2/1
  6x6 v-u_rotation/1(y) -> Demux/1
  18x18 v-u_rotation/1(y) -> m_out|a/1

== system FourRigidBarsAug/Bar #3 + revolute joint at C2=P3/Multi port rigid body ==
  in1 : Inport  PortDimensions=18
  in2 : Inport  Port=2  PortDimensions=6
  Demux : Demux  Outputs=[ 6 18]
  Gain : RCTblocks/Uncertain State Space  Tag=USS  USystem=uss(InvDynAug)  UValue=[]  X0=[]  uX0=[]
  Mux : Mux  Inputs=[ 18 6]
  out1 : Outport
  out2 : Outport  Port=2
  wires:
  Demux/2 -> out2/1
  in2/1 -> Mux/2
  Demux/1 -> out1/1
  in1/1 -> Mux/1
  Gain/1 -> Demux/1
  Mux/1 -> Gain/1

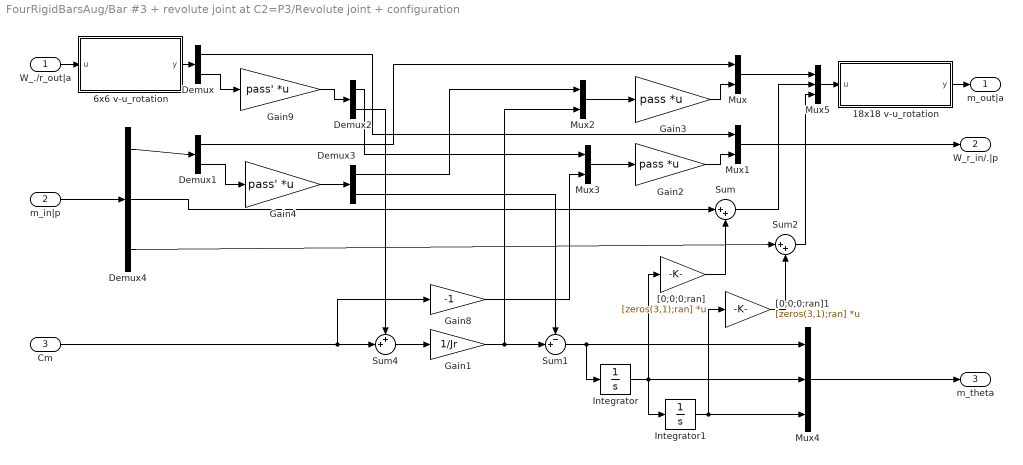
== system FourRigidBarsAug/Bar #3 + revolute joint at C2=P3/Revolute joint + configuration ==
  W_./r_out|a : Inport  PortDimensions=6
  m_in|p : Inport  Port=2  PortDimensions=18
  Cm : Inport  Port=3  PortDimensions=1
  18x18 v-u_rotation : Subsystem  mask(18x18 rotation matrix (around a given axis)){ra=ra, theta=theta, transp=on}
      mask prompts: ra "Rotation axis (3x1 vector)"; theta "Angle (rad)"; transp "Matrix transposed"
      mask help:
      | For 6 d.o.f. body motion vector (3 translations and 3 rotations, acceleration velocities and positions), this block Implement the 18x18 rotation matrix (or its transposed)  for a given angle around a given axis.
      |
      | Angle  (rad) can be an uncertain parameter declared with "ureal" with mode 'Range'
      | Ex: ureal('NAME',0,'Range',[-pi pi])
      | Then, ULINEARIZE will provide a model involving the block named "tan_NAME_div4".
      mask init:
      | vUrotation3x3
      mask Help: web('Doc6vurotation.html','-browser')
      mask Display:
      | disp('v-rot\n18x18')
      | if transp
      |     port_label('input', 1, '[.]_R1')
      |     port_label('output', 1, '[.]_R2')
      | else
      |     port_label('input', 1, '[.]_R2')
      |     port_label('output', 1, '[.]_R1')
      | end
  6x6 v-u_rotation : Subsystem  mask(6x6 rotation matrix (around a given axis)){ra=ra, theta=theta, transp=off}
      mask prompts: ra "Rotation axis (3x1 vector)"; theta "Angle (rad)"; transp "Matrix transposed"
      mask help:
      | For 6 d.o.f. body motion (3 translations and 3 rotations), this block Implement the 6x6 rotation matrix (or its transposed) for a given angle around a given axis.
      |
      | Angle  (rad) can be an uncertain parameter declared with "ureal" with mode 'Range'
      | Ex: ureal('NAME',0,'Range',[-pi pi])
      | Then, ULINEARIZE will provide a model involving the block named "tan_NAME_div4".
      mask init:
      | vUrotation3x3
      mask Help: web('Doc6vurotation.html','-browser')
      mask Display:
      | disp('v-rot\n6x6')
      | if transp
      |     port_label('input', 1, '[.]_R1')
      |     port_label('output', 1, '[.]_R2')
      | else
      |     port_label('input', 1, '[.]_R2')
      |     port_label('output', 1, '[.]_R1')
      | end
  Demux : Demux  Outputs=[3 3]
  Demux1 : Demux  Outputs=[3 3]
  Demux2 : Demux  Outputs=[2 1]
  Demux3 : Demux  Outputs=[2 1]
  Demux4 : Demux  Outputs=[6 6 6]
  Gain1 : Gain  Gain=1/Jr
  Gain2 : Gain  Gain=pass  Multiplication=Matrix(K*u) (u vector)
  Gain3 : Gain  Gain=pass  Multiplication=Matrix(K*u) (u vector)
  Gain4 : Gain  Gain=pass'  Multiplication=Matrix(K*u) (u vector)
  Gain8 : Gain  Gain=-1
  Gain9 : Gain  Gain=pass'  Multiplication=Matrix(K*u) (u vector)
  Integrator : Integrator
  Integrator1 : Integrator
  Mux : Mux  Inputs=[3 3]
  Mux1 : Mux  Inputs=[3 3]
  Mux2 : Mux  Inputs=[2 1]
  Mux3 : Mux  Inputs=[2 1]
  Mux4 : Mux  Inputs=3
  Mux5 : Mux  Inputs=[6 6 6]
  Sum : Sum  Inputs=|++
  Sum1 : Sum  Inputs=-+|
  Sum2 : Sum  Inputs=|++
  Sum4 : Sum  Inputs=++|
  "[0;0;0;ran]" : Gain  Gain=[zeros(3,1);ran]  Multiplication=Matrix(K*u) (u vector)
  "[0;0;0;ran]1" : Gain  Gain=[zeros(3,1);ran]  Multiplication=Matrix(K*u) (u vector)
  m_out|a : Outport  VectorParamsAs1DForOutWhenUnconnected=off
  W_r_in/.|p : Outport  Port=2  VectorParamsAs1DForOutWhenUnconnected=off
  m_theta : Outport  Port=3  VectorParamsAs1DForOutWhenUnconnected=off
  wires:
  18x18 v-u_rotation/1(y) -> m_out|a/1
  6x6 v-u_rotation/1(y) -> Demux/1
  Demux3/1 -> Mux2/1
  Demux2/1 -> Mux3/1
  Gain8/1 -> Mux3/2
  Mux3/1 -> Gain2/1
  Gain4/1 -> Demux3/1
  Demux1/2 -> Gain4/1
  Mux2/1 -> Gain3/1
  Demux2/2 -> Sum4/1
  Gain9/1 -> Demux2/1
  Demux3/2 -> Sum1/1
  Gain3/1 -> Mux/2
  Sum4/1 -> Gain1/1
  Gain1/1 -> Sum1/2, Mux2/2
  Demux/2 -> Gain9/1
  Gain2/1 -> Mux1/2
  Demux/1 -> Mux1/1
  Cm/1 -> Sum4/2, Gain8/1
  Demux1/1 -> Mux/1
  Mux1/1 -> W_r_in/.|p/1
  W_./r_out|a/1 -> 6x6 v-u_rotation/1(u)
  Demux4/1 -> Demux1/1
  m_in|p/1 -> Demux4/1
  Integrator/1 -> "[0;0;0;ran]"/1, Mux4/2, Integrator1/1
  Mux4/1 -> m_theta/1
  Sum1/1 -> Integrator/1, Mux4/1
  Integrator1/1 -> "[0;0;0;ran]1"/1, Mux4/3
  "[0;0;0;ran]"/1 -> Sum/2
  "[0;0;0;ran]1"/1 -> Sum2/2
  Demux4/2 -> Sum/1
  Demux4/3 -> Sum2/1
  Mux/1 -> Mux5/1
  Mux5/1 -> 18x18 v-u_rotation/1(u)
  Sum/1 -> Mux5/2
  Sum2/1 -> Mux5/3

== system FourRigidBarsAug/Bar #1 + revolute joint at P1/Revolute joint + configuration/18x18 v-u_rotation ==
  u : Inport  PortDimensions=18
  Demux : Demux  Outputs=[3 3 3 3 3 3]
  Mux : Mux  Inputs=[3 3 3 3 3 3]
  Subsystem : Subsystem
  Subsystem1 : Subsystem
  Subsystem2 : Subsystem
  Subsystem3 : Subsystem
  Subsystem4 : Subsystem
  Subsystem5 : Subsystem
  y : Outport  VectorParamsAs1DForOutWhenUnconnected=off
  wires:
  Subsystem1/1(Out1) -> Mux/2
  Subsystem/1(Out1) -> Mux/1
  Demux/2 -> Subsystem1/1(In1)
  Demux/1 -> Subsystem/1(In1)
  u/1 -> Demux/1
  Mux/1 -> y/1
  Demux/3 -> Subsystem2/1(In1)
  Subsystem2/1(Out1) -> Mux/3
  Demux/4 -> Subsystem3/1(In1)
  Subsystem3/1(Out1) -> Mux/4
  Demux/5 -> Subsystem4/1(In1)
  Subsystem4/1(Out1) -> Mux/5
  Demux/6 -> Subsystem5/1(In1)
  Subsystem5/1(Out1) -> Mux/6

== system FourRigidBarsAug/Bar #1 + revolute joint at P1/Revolute joint + configuration/6x6 v-u_rotation ==
  u : Inport  PortDimensions=6
  Demux : Demux  Outputs=[3 3]
  Mux : Mux  Inputs=[3 3]
  Subsystem : Subsystem
  Subsystem1 : Subsystem
  y : Outport  VectorParamsAs1DForOutWhenUnconnected=off
  wires:
  Mux/1 -> y/1
  u/1 -> Demux/1
  Demux/1 -> Subsystem/1(In1)
  Demux/2 -> Subsystem1/1(In1)
  Subsystem/1(Out1) -> Mux/1
  Subsystem1/1(Out1) -> Mux/2

== system FourRigidBarsAug/Bar #2 + revolute joint at C1=P2/Revolute joint + configuration/18x18 v-u_rotation ==
  u : Inport  PortDimensions=18
  Demux : Demux  Outputs=[3 3 3 3 3 3]
  Mux : Mux  Inputs=[3 3 3 3 3 3]
  Subsystem : Subsystem
  Subsystem1 : Subsystem
  Subsystem2 : Subsystem
  Subsystem3 : Subsystem
  Subsystem4 : Subsystem
  Subsystem5 : Subsystem
  y : Outport  VectorParamsAs1DForOutWhenUnconnected=off
  wires:
  Subsystem5/1(Out1) -> Mux/6
  Demux/6 -> Subsystem5/1(In1)
  Subsystem4/1(Out1) -> Mux/5
  Demux/5 -> Subsystem4/1(In1)
  Subsystem3/1(Out1) -> Mux/4
  Demux/4 -> Subsystem3/1(In1)
  Subsystem2/1(Out1) -> Mux/3
  Demux/3 -> Subsystem2/1(In1)
  Mux/1 -> y/1
  u/1 -> Demux/1
  Demux/1 -> Subsystem/1(In1)
  Demux/2 -> Subsystem1/1(In1)
  Subsystem/1(Out1) -> Mux/1
  Subsystem1/1(Out1) -> Mux/2

== system FourRigidBarsAug/Bar #2 + revolute joint at C1=P2/Revolute joint + configuration/6x6 v-u_rotation ==
  u : Inport  PortDimensions=6
  Demux : Demux  Outputs=[3 3]
  Mux : Mux  Inputs=[3 3]
  Subsystem : Subsystem
  Subsystem1 : Subsystem
  y : Outport  VectorParamsAs1DForOutWhenUnconnected=off
  wires:
  Subsystem1/1(Out1) -> Mux/2
  Subsystem/1(Out1) -> Mux/1
  Demux/2 -> Subsystem1/1(In1)
  Demux/1 -> Subsystem/1(In1)
  u/1 -> Demux/1
  Mux/1 -> y/1

== system FourRigidBarsAug/Bar #3 + revolute joint at C2=P3/Revolute joint + configuration/18x18 v-u_rotation ==
  u : Inport  PortDimensions=18
  Demux : Demux  Outputs=[3 3 3 3 3 3]
  Mux : Mux  Inputs=[3 3 3 3 3 3]
  Subsystem : Subsystem
  Subsystem1 : Subsystem
  Subsystem2 : Subsystem
  Subsystem3 : Subsystem
  Subsystem4 : Subsystem
  Subsystem5 : Subsystem
  y : Outport  VectorParamsAs1DForOutWhenUnconnected=off
  wires:
  Subsystem1/1(Out1) -> Mux/2
  Subsystem/1(Out1) -> Mux/1
  Demux/2 -> Subsystem1/1(In1)
  Demux/1 -> Subsystem/1(In1)
  u/1 -> Demux/1
  Mux/1 -> y/1
  Demux/3 -> Subsystem2/1(In1)
  Subsystem2/1(Out1) -> Mux/3
  Demux/4 -> Subsystem3/1(In1)
  Subsystem3/1(Out1) -> Mux/4
  Demux/5 -> Subsystem4/1(In1)
  Subsystem4/1(Out1) -> Mux/5
  Demux/6 -> Subsystem5/1(In1)
  Subsystem5/1(Out1) -> Mux/6

== system FourRigidBarsAug/Bar #3 + revolute joint at C2=P3/Revolute joint + configuration/6x6 v-u_rotation ==
  u : Inport  PortDimensions=6
  Demux : Demux  Outputs=[3 3]
  Mux : Mux  Inputs=[3 3]
  Subsystem : Subsystem
  Subsystem1 : Subsystem
  y : Outport  VectorParamsAs1DForOutWhenUnconnected=off
  wires:
  Mux/1 -> y/1
  u/1 -> Demux/1
  Demux/1 -> Subsystem/1(In1)
  Demux/2 -> Subsystem1/1(In1)
  Subsystem/1(Out1) -> Mux/1
  Subsystem1/1(Out1) -> Mux/2

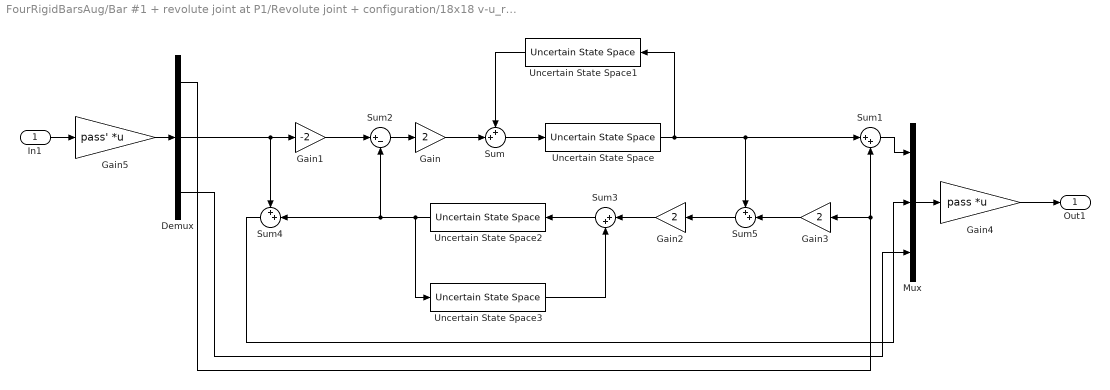
== system FourRigidBarsAug/Bar #1 + revolute joint at P1/Revolute joint + configuration/18x18 v-u_rotation/Subsystem ==
  In1 : Inport
  Demux : Demux  Outputs=3
  Gain : Gain  Gain=2
  Gain1 : Gain  Gain=-2
  Gain2 : Gain  Gain=2
  Gain3 : Gain  Gain=2
  Gain4 : Gain  Gain=pass  Multiplication=Matrix(K*u) (u vector)
  Gain5 : Gain  Gain=pass'  Multiplication=Matrix(K*u) (u vector)
  Mux : Mux  Inputs=3
  Sum : Sum  Inputs=++|
  Sum1 : Sum  Inputs=|++
  Sum2 : Sum  Inputs=|+-
  Sum3 : Sum  Inputs=|++
  Sum4 : Sum  Inputs=++|
  Sum5 : Sum  Inputs=++|
  Uncertain State Space{,1..3} (4 alike) : RCTblocks/Uncertain State Space  Tag=USS  USystem=uss(sig4)  UValue=[]  X0=[]  uX0=[]
  Out1 : Outport  VectorParamsAs1DForOutWhenUnconnected=off
  wires:
  Gain5/1 -> Demux/1
  Gain4/1 -> Out1/1
  Uncertain State Space3/1 -> Sum3/2
  Gain2/1 -> Sum3/1
  In1/1 -> Gain5/1
  Gain/1 -> Sum/2
  Uncertain State Space2/1 -> Uncertain State Space3/1, Sum4/2, Sum2/2
  Demux/1 -> Gain3/1, Sum1/2
  Demux/3 -> Mux/3
  Mux/1 -> Gain4/1
  Sum4/1 -> Mux/2
  Sum3/1 -> Uncertain State Space2/1
  Gain1/1 -> Sum2/1
  Uncertain State Space/1 -> Uncertain State Space1/1, Sum5/1, Sum1/1
  Gain3/1 -> Sum5/2
  Sum/1 -> Uncertain State Space/1
  Demux/2 -> Sum4/1, Gain1/1
  Uncertain State Space1/1 -> Sum/1
  Sum2/1 -> Gain/1
  Sum1/1 -> Mux/1
  Sum5/1 -> Gain2/1

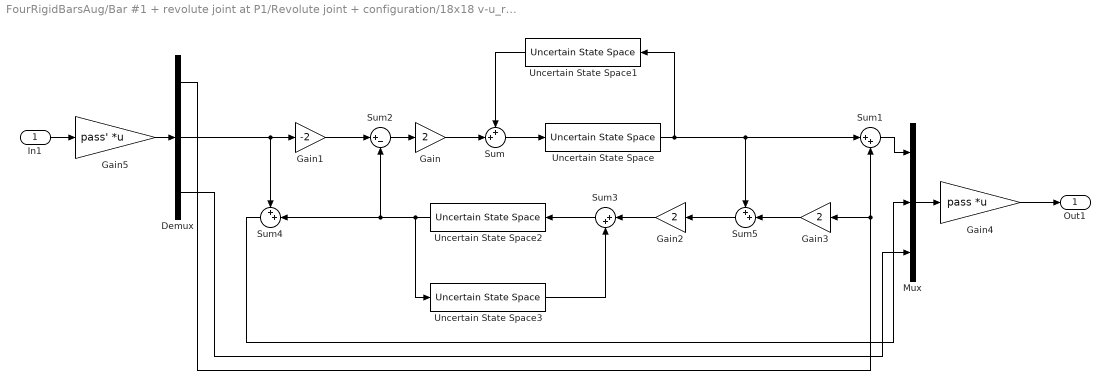
== system FourRigidBarsAug/Bar #1 + revolute joint at P1/Revolute joint + configuration/18x18 v-u_rotation/Subsystem1 ==
  In1 : Inport
  Demux : Demux  Outputs=3
  Gain : Gain  Gain=2
  Gain1 : Gain  Gain=-2
  Gain2 : Gain  Gain=2
  Gain3 : Gain  Gain=2
  Gain4 : Gain  Gain=pass  Multiplication=Matrix(K*u) (u vector)
  Gain5 : Gain  Gain=pass'  Multiplication=Matrix(K*u) (u vector)
  Mux : Mux  Inputs=3
  Sum : Sum  Inputs=++|
  Sum1 : Sum  Inputs=|++
  Sum2 : Sum  Inputs=|+-
  Sum3 : Sum  Inputs=|++
  Sum4 : Sum  Inputs=++|
  Sum5 : Sum  Inputs=++|
  Uncertain State Space{,1..3} (4 alike) : RCTblocks/Uncertain State Space  Tag=USS  USystem=uss(sig4)  UValue=[]  X0=[]  uX0=[]
  Out1 : Outport  VectorParamsAs1DForOutWhenUnconnected=off
  wires:
  Gain5/1 -> Demux/1
  Sum5/1 -> Gain2/1
  Sum1/1 -> Mux/1
  Sum2/1 -> Gain/1
  Uncertain State Space1/1 -> Sum/1
  Demux/2 -> Gain1/1, Sum4/1
  Sum/1 -> Uncertain State Space/1
  Gain3/1 -> Sum5/2
  Uncertain State Space/1 -> Sum1/1, Sum5/1, Uncertain State Space1/1
  Gain1/1 -> Sum2/1
  Sum3/1 -> Uncertain State Space2/1
  Sum4/1 -> Mux/2
  Mux/1 -> Gain4/1
  Demux/3 -> Mux/3
  Demux/1 -> Sum1/2, Gain3/1
  Uncertain State Space2/1 -> Sum2/2, Sum4/2, Uncertain State Space3/1
  Gain/1 -> Sum/2
  In1/1 -> Gain5/1
  Gain2/1 -> Sum3/1
  Uncertain State Space3/1 -> Sum3/2
  Gain4/1 -> Out1/1
